simulink model "ESP32Arm5DOF"  (R2024a)
settings: Solver=VariableStepAuto  StartTime=0.0  StopTime=10.0  RelTol=1e-3
libraries: arduinolib x5, SignalEditorBlockLib x5, arduinosensorlib x1
settings Model: Creator=Akbar  LastModifiedBy=Akbar

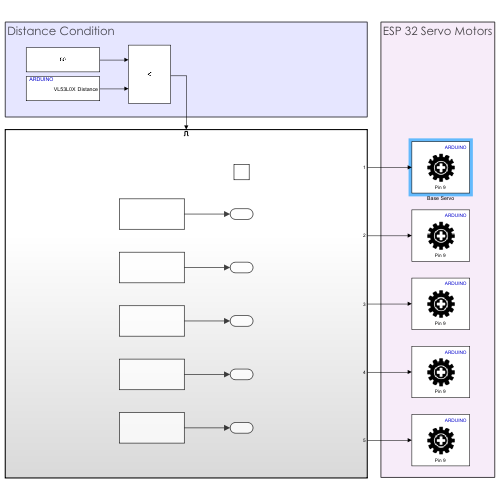
[thumbnail: Simulink's stored preview of the top-level diagram]
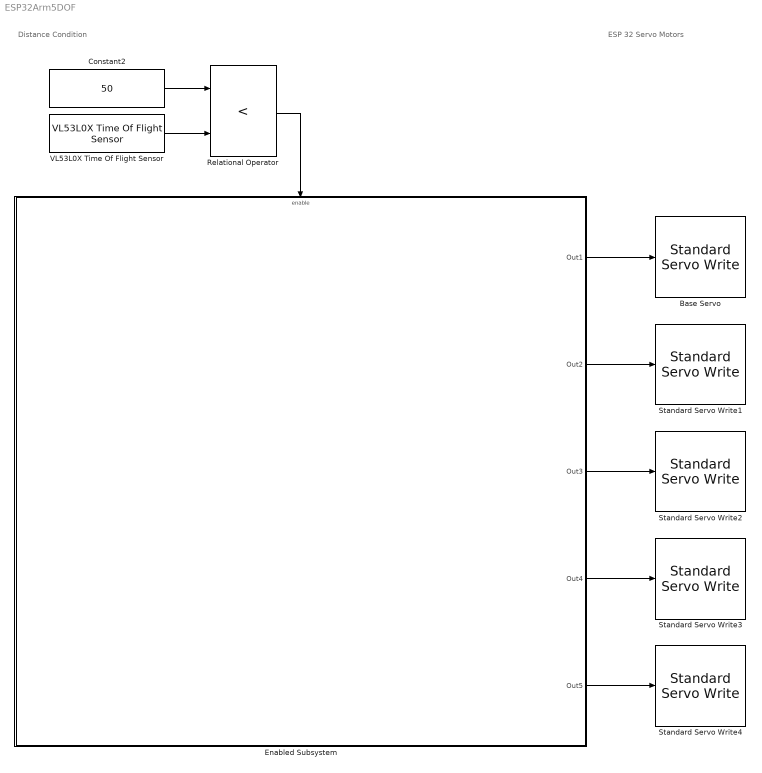
== system ESP32Arm5DOF ==
  note: Distance Condition
  note: ESP 32 Servo Motors
  Base Servo : arduinolib/Standard Servo Write  pinNumber=9  ServoIndex=0  blockPlatform=ARDUINO
  Constant2 : Constant  Value=50
  Enabled Subsystem : Subsystem  TreatAsAtomicUnit=on
  Relational Operator : RelationalOperator  Operator=<  OutDataTypeStr=boolean  RndMeth=Simplest  InputSameDT=off
  Standard Servo Write{1..4} (4 alike) : arduinolib/Standard Servo Write  pinNumber=9  ServoIndex=0  blockPlatform=ARDUINO
  VL53L0X Time Of Flight Sensor : arduinosensorlib/VL53L0X Time Of Flight Sensor  I2CModule=0  I2CAddress=0x29  BitRate=1000000  RangingMode=Default  SampleTime=-1
  wires:
  VL53L0X Time Of Flight Sensor/1 -> Relational Operator/2
  Constant2/1 -> Relational Operator/1
  Enabled Subsystem/3(Out3) -> Standard Servo Write2/1
  Enabled Subsystem/5(Out5) -> Standard Servo Write4/1
  Enabled Subsystem/1(Out1) -> Base Servo/1
  Enabled Subsystem/4(Out4) -> Standard Servo Write3/1
  Enabled Subsystem/2(Out2) -> Standard Servo Write1/1
  Relational Operator/1 -> Enabled Subsystem/Enable

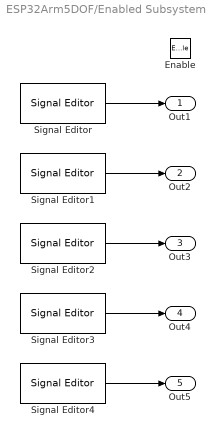
== system ESP32Arm5DOF/Enabled Subsystem ==
  Enable : EnablePort
  Signal Editor{,1..4} (5 alike) : SignalEditorBlockLib/Signal Editor  FileName=untitled.mat  ActiveScenario=Scenario  ActiveSignal=Signal 1  IsBus=off  OutputBusObjectStr=Bus: BusObject  SampleTime=0  Interpolate=off  ZeroCross=off  OutputAfterFinalValue=Setting to zero  Unit=inherit  PreserveSignalName=on  ApplySigPropsToAllScenarios=on  ApplySigPropsToAllSignals=off
  Out1 : Outport
  Out2 : Outport  Port=2
  Out3 : Outport  Port=3
  Out4 : Outport  Port=4
  Out5 : Outport  Port=5
  wires:
  Signal Editor/1 -> Out1/1
  Signal Editor1/1 -> Out2/1
  Signal Editor2/1 -> Out3/1
  Signal Editor3/1 -> Out4/1
  Signal Editor4/1 -> Out5/1
